simulink model "VDC_TEST_VERNIS"  (R2023b)
settings: Solver=FixedStepAuto  StartTime=0.0  StopTime=10.0  RelTol=1e-3
libraries: simulink x3
settings Model: Creator=no  LastModifiedBy=no
settings OptimizationCC: DefaultParameterBehavior=Inlined
settings RTWCC: Description=INTECRIO Real-Time Target  SystemTargetFile=irt.tlc  TemplateMakefile=irt_default_tmf
settings STFCustomTargetCC: UtilityFuncGeneration=Shared location  MatFileLogging=on  GRTInterface=on  SystemTargetFile=irt.tlc
settings GRTTargetCC: UtilityFuncGeneration=Shared location  ParMdlRefBuildCompliant=off  CompOptLevelCompliant=off  ConcurrentExecutionCompliant=off  CombineOutputUpdateFcns=off  CPPClassGenCompliant=off  GRTInterface=on  UseToolchainInfoCompliant=off  GenerateASAP2=on

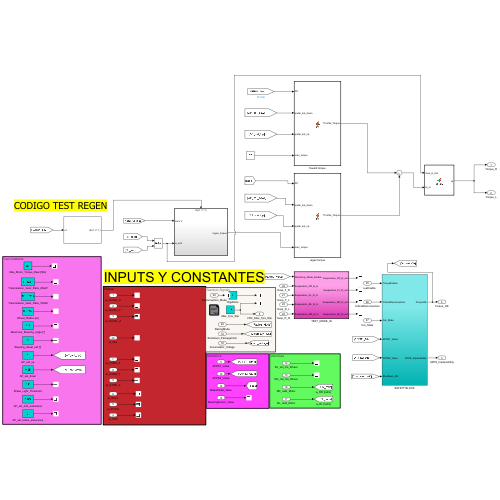
[thumbnail: Simulink's stored preview of the top-level diagram]
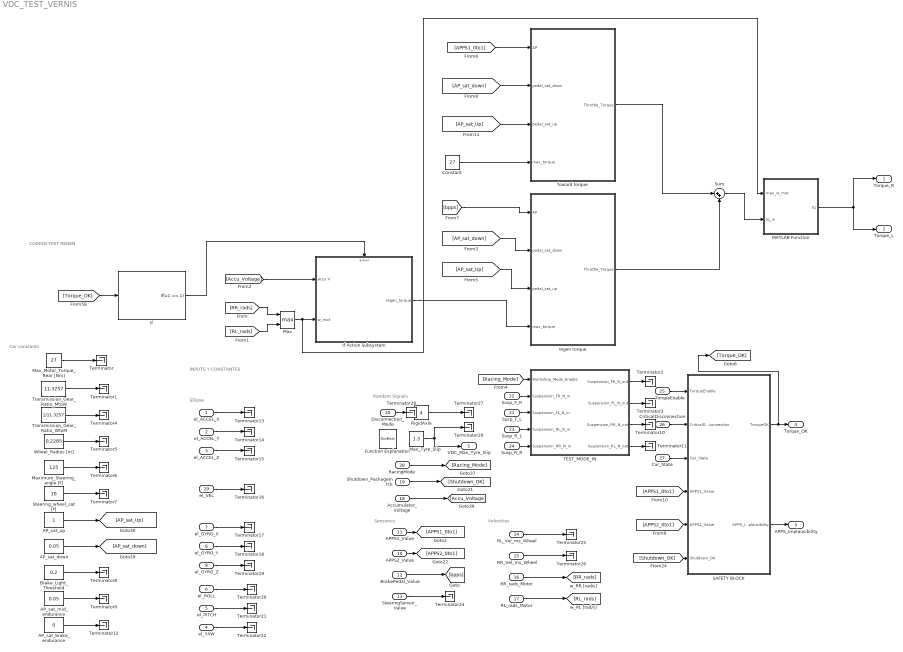
== system VDC_TEST_VERNIS ==
  note: CODIGO TEST REGEN
  note: INPUTS Y CONSTANTES
  note: Ellipse
  note: Sensorics
  note: Velocities
  note: Car constants
  note: Random Signals
  el_ACCEL_X : Inport
  el_ACCEL_Y : Inport  Port=2
  el_ACCEL_Z : Inport  Port=3
  el_YAW : Inport  Port=4
  el_PITCH : Inport  Port=5
  el_ROLL : Inport  Port=6
  el_GYRO_X : Inport  Port=7
  el_GYRO_Y : Inport  Port=8
  el_GYRO_Z : Inport  Port=9
  APPS2_Value : Inport  Port=10
  APPS1_Value : Inport  Port=11
  BrakePedal_Value : Inport  Port=12
  SteeringSensor_Value : Inport  Port=13
  RL_Vel_ms_Wheel : Inport  Port=14
  RR_Vel_ms_Wheel : Inport  Port=15
  RR_rads_Motor : Inport  Port=16
  RL_rads_Motor : Inport  Port=17
  Accumulator_Voltage : Inport  Port=18
  Shutdown_PackageIntck : Inport  Port=19
  Disconnection_Mode : Inport  Port=20
  Susp_F_L : Inport  Port=21
  Susp_F_R : Inport  Port=22
  Susp_R_L : Inport  Port=23
  Susp_R_R : Inport  Port=24
  TorqueEnable : Inport  Port=25
  CriticalDisconnection : Inport  Port=26
  Car_State : Inport  Port=27
  RacingMode : Inport  Port=28
  el_VEL : Inport  Port=29
  AP_sat_brake_endurance : Constant  Value=0
  AP_sat_down : Constant  Value=0.05
  AP_sat_mid_endurance : Constant  Value=0.05
  AP_sat_up : Constant
  Brake_Light_Threshold : Constant  Value=0.2
  Constant : Constant  Value=27
  Function Explanation : simulink/Model-Wide Utilities/DocBlock  DocumentType=Text
      content=|
      | Comparing the speed of the Ellipse and the speed of the Wheels, we can
      | determine the % of deviation between both (which is the slip). With
      | calculations from the Tyres & Performance Department, we know that the
      | maximum optimal slip in a STRAIGHT line is 15%. Therefore (using the Magic
      | Formula), we can determine the maximum X-Force permissible by the Wheels
      | with that % of slip (which is the constant Max_Fx_Tyre, input
      | of Rigid Axle).
      |
      | With that and the radius of the Wheels, we can calculate the maximum
      | Torque for it to stop slipping.
  If : If  IfExpression=u1 == 1  ShowElse=off
  If Action Subsystem : Subsystem  TreatAsAtomicUnit=on
  MATLAB Function : MATLAB Function  TreatAsAtomicUnit=on
  Max : MinMax  Function=max  Inputs=2
  Max_Motor_Torque_Rear [Nm] : Constant  Value=27
  Max_Tyre_Slip : Constant  Value=1.3
  Maximum_Steering_angle [º] : Constant  Value=125
  RigidAxle : Constant  Value=4
  SAFETY BLOCK : Subsystem
  Steering_wheel_sat [º] : Constant  Value=10
  Sum : Sum  Inputs=|++
  TEST_MODE_IN : Subsystem  TreatAsAtomicUnit=on
  Terminator{,1..22,24..29} (29 alike) : Terminator
  Transmission_Gear_Ratio_MtoW : Constant  Value=11.3257
  Transmission_Gear_Ratio_WtoM : Constant  Value=1/11.3257
  Wheel_Radius [m] : Constant  Value=0.2285
  foward torque : MATLAB Function  TreatAsAtomicUnit=on
  regen torque : MATLAB Function  TreatAsAtomicUnit=on
  Torque_R : Outport
  Torque_L : Outport  Port=2
  APPS_Implausibility : Outport  Port=3  VectorParamsAs1DForOutWhenUnconnected=off
  Torque_OK : Outport  Port=4  VectorParamsAs1DForOutWhenUnconnected=off
  VDC_Max_Tyre_Slip : Outport  Port=5
  wires:
  SteeringSensor_Value/1 -> Terminator24/1
  APPS1_Value/1 -> [APPS1_0to1]
  BrakePedal_Value/1 -> [bpps]
  APPS2_Value/1 -> [APPS2_0to1]
  Transmission_Gear_Ratio_MtoW/1 -> Terminator1/1
  Transmission_Gear_Ratio_WtoM/1 -> Terminator4/1
  Wheel_Radius [m]/1 -> Terminator5/1
  Max_Motor_Torque_Rear [Nm]/1 -> Terminator/1
  Shutdown_PackageIntck/1 -> [Shutdown_OK]
  Accumulator_Voltage/1 -> [Accu_Voltage]
  Maximum_Steering_angle [º]/1 -> Terminator6/1
  Steering_wheel_sat [º]/1 -> Terminator7/1
  [Racing_Mode] -> TEST_MODE_IN/1(Workshop_Mode_Enable)
  Susp_F_R/1 -> TEST_MODE_IN/2(Suspension_FR_N_in)
  Susp_R_L/1 -> TEST_MODE_IN/4(Suspension_RL_N_in)
  Susp_R_R/1 -> TEST_MODE_IN/5(Suspension_RR_N_in)
  Susp_F_L/1 -> TEST_MODE_IN/3(Suspension_FL_N_in)
  Max_Tyre_Slip/1 -> Terminator29/1, VDC_Max_Tyre_Slip/1
  CriticalDisconnection/1 -> SAFETY BLOCK/2(CriticalDisconnection)
  TorqueEnable/1 -> SAFETY BLOCK/1(TorqueEnable)
  SAFETY BLOCK/1(TorqueOK) -> Torque_OK/1, [Torque_OK]
  [APPS1_0to1] -> SAFETY BLOCK/4(APPS1_Value)
  SAFETY BLOCK/2(APPS_Implausibility) -> APPS_Implausibility/1
  [APPS2_0to1] -> SAFETY BLOCK/5(APPS2_Value)
  [Shutdown_OK] -> SAFETY BLOCK/6(Shutdown_OK)
  Car_State/1 -> SAFETY BLOCK/3(Car_State)
  AP_sat_up/1 -> [AP_sat_Up]
  AP_sat_down/1 -> [AP_sat_down]
  TEST_MODE_IN/2(Suspension_FL_N_out) -> Terminator3/1
  TEST_MODE_IN/4(Suspension_RL_N_out) -> Terminator11/1
  TEST_MODE_IN/3(Suspension_RR_N_out) -> Terminator10/1
  TEST_MODE_IN/1(Suspension_FR_N_out) -> Terminator2/1
  RacingMode/1 -> [Racing_Mode]
  RL_rads_Motor/1 -> [RL_rads]
  RR_rads_Motor/1 -> [RR_rads]
  RR_Vel_ms_Wheel/1 -> Terminator26/1
  RL_Vel_ms_Wheel/1 -> Terminator25/1
  Brake_Light_Threshold/1 -> Terminator8/1
  AP_sat_mid_endurance/1 -> Terminator9/1
  AP_sat_brake_endurance/1 -> Terminator12/1
  RigidAxle/1 -> Terminator27/1
  [Torque_OK] -> If/1
  If/1 -> If Action Subsystem/Action
  [Accu_Voltage] -> If Action Subsystem/1(accu V)
  [RR_rads] -> Max/1
  [RL_rads] -> Max/2
  Max/1 -> MATLAB Function/1(max_w_mot), If Action Subsystem/2(w_mot)
  If Action Subsystem/1(regen_torque) -> regen torque/4(max_torque)
  el_ACCEL_Z/1 -> Terminator15/1
  el_ACCEL_Y/1 -> Terminator14/1
  el_ACCEL_X/1 -> Terminator13/1
  el_VEL/1 -> Terminator16/1
  el_GYRO_Z/1 -> Terminator19/1
  el_GYRO_Y/1 -> Terminator18/1
  el_GYRO_X/1 -> Terminator17/1
  el_PITCH/1 -> Terminator21/1
  el_ROLL/1 -> Terminator20/1
  el_YAW/1 -> Terminator22/1
  Disconnection_Mode/1 -> Terminator28/1
  [APPS1_0to1] -> foward torque/1(AP)
  [bpps] -> regen torque/1(AP)
  [AP_sat_Up] -> regen torque/3(pedal_sat_up)
  [AP_sat_down] -> regen torque/2(pedal_sat_down)
  [AP_sat_down] -> foward torque/2(pedal_sat_down)
  [AP_sat_Up] -> foward torque/3(pedal_sat_up)
  Constant/1 -> foward torque/4(max_torque)
  foward torque/1(Throttle_Torque) -> Sum/1
  regen torque/1(Throttle_Torque) -> Sum/2
  Sum/1 -> MATLAB Function/2(tq_in)
  MATLAB Function/1(tq) -> Torque_L/1, Torque_R/1

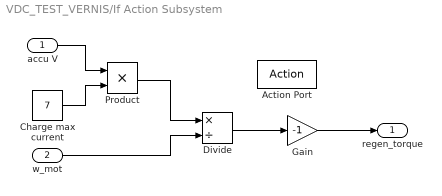
== system VDC_TEST_VERNIS/If Action Subsystem ==
  accu V : Inport
  w_mot : Inport  Port=2
  Action Port : ActionPort  ActionPortLabel=if(u1 == 1)
  Charge max current : Constant  Value=7
  Divide : Product  Inputs=*/
  Gain : Gain  Gain=-1
  Product : Product
  regen_torque : Outport
  wires:
  Gain/1 -> regen_torque/1
  Charge max current/1 -> Product/2
  w_mot/1 -> Divide/2
  Divide/1 -> Gain/1
  accu V/1 -> Product/1
  Product/1 -> Divide/1

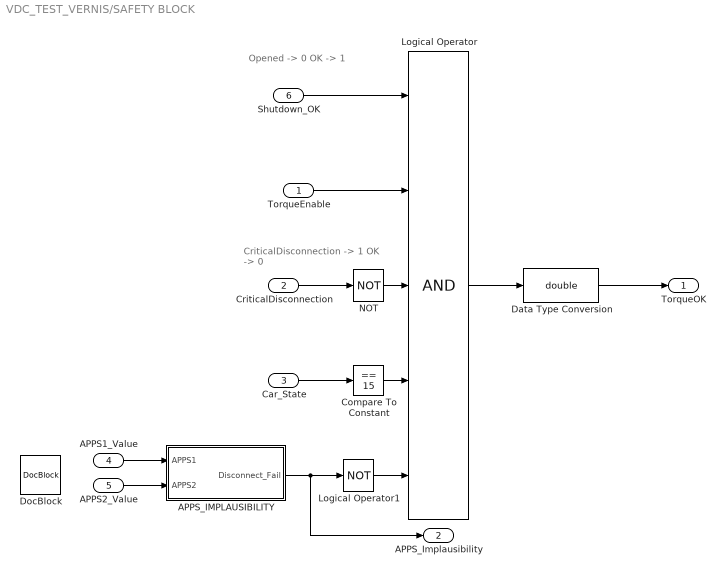
== system VDC_TEST_VERNIS/SAFETY BLOCK ==
  note: CriticalDisconnection -> 1
      | OK -> 0
  note: Opened -> 0
      | OK -> 1
  TorqueEnable : Inport
  CriticalDisconnection : Inport  Port=2
  Car_State : Inport  Port=3
  APPS1_Value : Inport  Port=4
  APPS2_Value : Inport  Port=5
  Shutdown_OK : Inport  Port=6
  APPS_IMPLAUSIBILITY : Subsystem
  Compare To Constant : simulink/Logic and Bit Operations/Compare To Constant  relop===  const=15  OutDataTypeStr=boolean
  Data Type Conversion : DataTypeConversion  OutDataTypeStr=double  SaturateOnIntegerOverflow=off  RndMeth=Floor
  DocBlock : simulink/Model-Wide Utilities/DocBlock  DocumentType=Text
      content=|
      | Formula Student Rules 2024 -> T11.8.8
      |     If an implausibility occurs between the values of the APPSs and
      |     persists for more than 100 ms:
      |     • [EV ONLY] The power to the motor(s) must be immediately shut down
      |     completely. It is not necessary to completely deactivate the TS, the
      |     motor controller(s) shutting down the power to the motor(s) is
      |     sufficient.
      |
      | The 'Number_of_Periods' constant, if there's an Implausability, outputs the error X
      | periods (100ms) after the Implausibility happened (25ms * X = 100ms).
  Logical Operator : Logic  Inputs=5  OutDataTypeStr=boolean
  Logical Operator1 : Logic  Operator=NOT  IconShape=distinctive  AllPortsSameDT=off  OutDataTypeStr=boolean
  NOT : Logic  Operator=NOT  IconShape=distinctive  AllPortsSameDT=off  OutDataTypeStr=boolean
  TorqueOK : Outport  VectorParamsAs1DForOutWhenUnconnected=off
  APPS_Implausibility : Outport  Port=2  VectorParamsAs1DForOutWhenUnconnected=off
  wires:
  Logical Operator/1 -> Data Type Conversion/1
  Car_State/1 -> Compare To Constant/1
  NOT/1 -> Logical Operator/3
  CriticalDisconnection/1 -> NOT/1
  TorqueEnable/1 -> Logical Operator/2
  APPS2_Value/1 -> APPS_IMPLAUSIBILITY/2(APPS2)
  APPS1_Value/1 -> APPS_IMPLAUSIBILITY/1(APPS1)
  APPS_IMPLAUSIBILITY/1(Disconnect_Fail) -> APPS_Implausibility/1, Logical Operator1/1
  Compare To Constant/1 -> Logical Operator/4
  Shutdown_OK/1 -> Logical Operator/1
  Logical Operator1/1 -> Logical Operator/5
  Data Type Conversion/1 -> TorqueOK/1

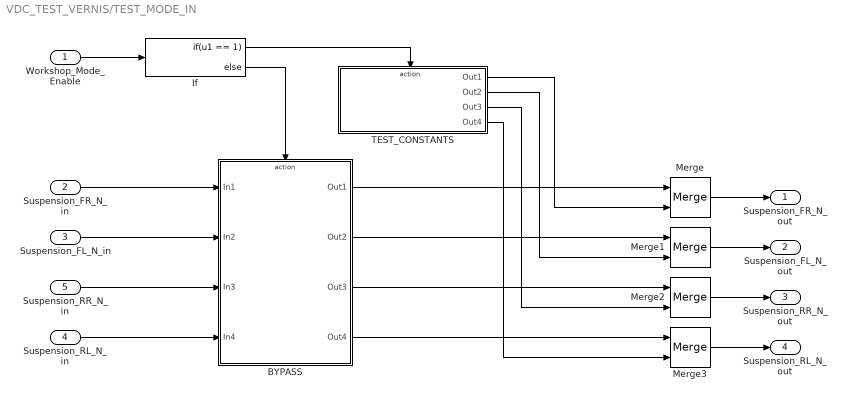
== system VDC_TEST_VERNIS/TEST_MODE_IN ==
  Workshop_Mode_Enable : Inport
  Suspension_FR_N_in : Inport  Port=2
  Suspension_FL_N_in : Inport  Port=3
  Suspension_RL_N_in : Inport  Port=4
  Suspension_RR_N_in : Inport  Port=5
  BYPASS : Subsystem  TreatAsAtomicUnit=on
  If : If  IfExpression=u1 == 1
  Merge{,1..3} (4 alike) : Merge
  TEST_CONSTANTS : Subsystem  TreatAsAtomicUnit=on
  Suspension_FR_N_out : Outport  VectorParamsAs1DForOutWhenUnconnected=off
  Suspension_FL_N_out : Outport  Port=2  VectorParamsAs1DForOutWhenUnconnected=off
  Suspension_RR_N_out : Outport  Port=3  VectorParamsAs1DForOutWhenUnconnected=off
  Suspension_RL_N_out : Outport  Port=4  VectorParamsAs1DForOutWhenUnconnected=off
  wires:
  Suspension_FR_N_in/1 -> BYPASS/1(In1)
  Suspension_FL_N_in/1 -> BYPASS/2(In2)
  Suspension_RR_N_in/1 -> BYPASS/3(In3)
  Suspension_RL_N_in/1 -> BYPASS/4(In4)
  Merge/1 -> Suspension_FR_N_out/1
  Merge1/1 -> Suspension_FL_N_out/1
  Merge2/1 -> Suspension_RR_N_out/1
  Merge3/1 -> Suspension_RL_N_out/1
  BYPASS/1(Out1) -> Merge/1
  BYPASS/2(Out2) -> Merge1/1
  BYPASS/3(Out3) -> Merge2/1
  BYPASS/4(Out4) -> Merge3/1
  Workshop_Mode_Enable/1 -> If/1
  If/2 -> BYPASS/Action
  If/1 -> TEST_CONSTANTS/Action
  TEST_CONSTANTS/4(Out4) -> Merge3/2
  TEST_CONSTANTS/3(Out3) -> Merge2/2
  TEST_CONSTANTS/2(Out2) -> Merge1/2
  TEST_CONSTANTS/1(Out1) -> Merge/2

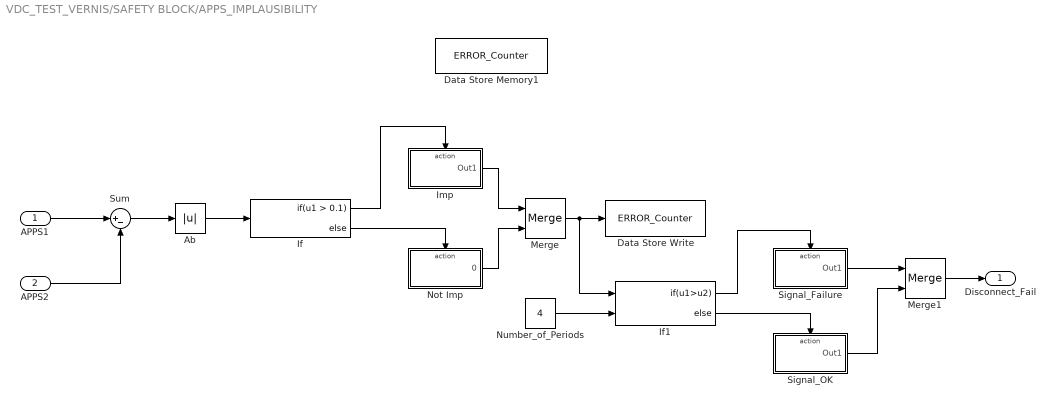
== system VDC_TEST_VERNIS/SAFETY BLOCK/APPS_IMPLAUSIBILITY ==
  APPS1 : Inport
  APPS2 : Inport  Port=2
  Ab : Abs  SaturateOnIntegerOverflow=off
  Data Store Memory1 : DataStoreMemory  DataStoreName=ERROR_Counter  ReadBeforeWriteMsg=warning  WriteAfterWriteMsg=warning  WriteAfterReadMsg=warning  ShowAdditionalParam=off
  Data Store Write : DataStoreWrite  DataStoreName=ERROR_Counter  IndexOptions=Index vector (dialog)  Indices=1  OutputSizes=1
  If : If  IfExpression=u1 > 0.1
  If1 : If  NumInputs=2  IfExpression=u1>u2
  Imp : Subsystem  TreatAsAtomicUnit=on
  Merge : Merge
  Merge1 : Merge
  Not Imp : Subsystem  TreatAsAtomicUnit=on
  Number_of_Periods : Constant  Value=4
  Signal_Failure : Subsystem  TreatAsAtomicUnit=on
  Signal_OK : Subsystem  TreatAsAtomicUnit=on
  Sum : Sum  Inputs=|+-
  Disconnect_Fail : Outport  VectorParamsAs1DForOutWhenUnconnected=off
  wires:
  Number_of_Periods/1 -> If1/2
  Imp/1(Out1) -> Merge/1
  Signal_Failure/1(Out1) -> Merge1/1
  Signal_OK/1(Out1) -> Merge1/2
  Merge1/1 -> Disconnect_Fail/1
  APPS1/1 -> Sum/1
  If/1 -> Imp/Action
  If1/2 -> Signal_OK/Action
  Merge/1 -> Data Store Write/1, If1/1
  If1/1 -> Signal_Failure/Action
  APPS2/1 -> Sum/2
  Ab/1 -> If/1
  If/2 -> Not Imp/Action
  Sum/1 -> Ab/1
  Not Imp/1(0) -> Merge/2

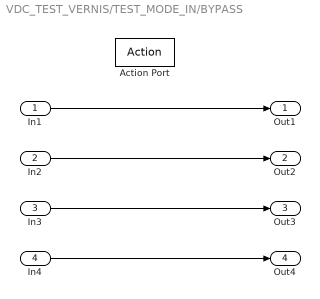
== system VDC_TEST_VERNIS/TEST_MODE_IN/BYPASS ==
  In1 : Inport
  In2 : Inport  Port=2
  In3 : Inport  Port=3
  In4 : Inport  Port=4
  Action Port : ActionPort  ActionPortLabel=else
  Out1 : Outport  VectorParamsAs1DForOutWhenUnconnected=off
  Out2 : Outport  Port=2  VectorParamsAs1DForOutWhenUnconnected=off
  Out3 : Outport  Port=3  VectorParamsAs1DForOutWhenUnconnected=off
  Out4 : Outport  Port=4  VectorParamsAs1DForOutWhenUnconnected=off
  wires:
  In1/1 -> Out1/1
  In2/1 -> Out2/1
  In3/1 -> Out3/1
  In4/1 -> Out4/1

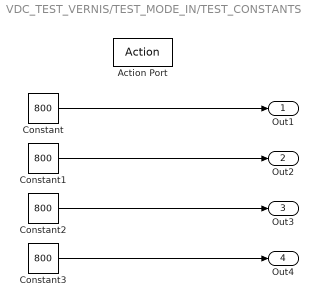
== system VDC_TEST_VERNIS/TEST_MODE_IN/TEST_CONSTANTS ==
  Action Port : ActionPort  ActionPortLabel=if(u1 == 1)
  Constant{,1..3} (4 alike) : Constant  Value=800
  Out1 : Outport  VectorParamsAs1DForOutWhenUnconnected=off
  Out2 : Outport  Port=2  VectorParamsAs1DForOutWhenUnconnected=off
  Out3 : Outport  Port=3  VectorParamsAs1DForOutWhenUnconnected=off
  Out4 : Outport  Port=4  VectorParamsAs1DForOutWhenUnconnected=off
  wires:
  Constant/1 -> Out1/1
  Constant1/1 -> Out2/1
  Constant2/1 -> Out3/1
  Constant3/1 -> Out4/1

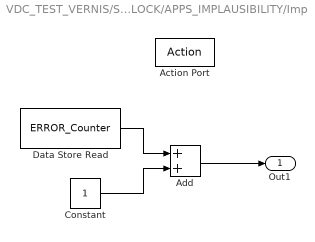
== system VDC_TEST_VERNIS/SAFETY BLOCK/APPS_IMPLAUSIBILITY/Imp ==
  Action Port : ActionPort  ActionPortLabel=if(u1 > 0.1)
  Add : Sum
  Constant : Constant  OutDataTypeStr=boolean
  Data Store Read : DataStoreRead  DataStoreName=ERROR_Counter  IndexOptions=Index vector (dialog)  Indices=1  OutputSizes=1
  Out1 : Outport  VectorParamsAs1DForOutWhenUnconnected=off
  wires:
  Data Store Read/1 -> Add/1
  Constant/1 -> Add/2
  Add/1 -> Out1/1

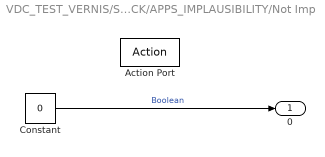
== system VDC_TEST_VERNIS/SAFETY BLOCK/APPS_IMPLAUSIBILITY/Not Imp ==
  Action Port : ActionPort  ActionPortLabel=else
  Constant : Constant  Value=0  OutDataTypeStr=double
  0 : Outport  VectorParamsAs1DForOutWhenUnconnected=off
  wires:
  Constant/1 -> 0/1  "Boolean"

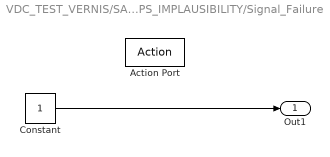
== system VDC_TEST_VERNIS/SAFETY BLOCK/APPS_IMPLAUSIBILITY/Signal_Failure ==
  Action Port : ActionPort  ActionPortLabel=if(u1>u2)
  Constant : Constant
  Out1 : Outport  VectorParamsAs1DForOutWhenUnconnected=off
  wires:
  Constant/1 -> Out1/1

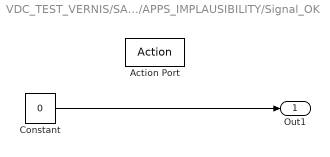
== system VDC_TEST_VERNIS/SAFETY BLOCK/APPS_IMPLAUSIBILITY/Signal_OK ==
  Action Port : ActionPort  ActionPortLabel=else
  Constant : Constant  Value=0
  Out1 : Outport  VectorParamsAs1DForOutWhenUnconnected=off
  wires:
  Constant/1 -> Out1/1

== matlab function VDC_TEST_VERNIS/foward torque ==
  data: Throttle_Torque output; AP input; pedal_sat_down input; pedal_sat_up input; max_torque input
function Throttle_Torque  = TT(AP, pedal_sat_down, pedal_sat_up, max_torque)
    if AP <= pedal_sat_down  
        Throttle_Response = 0;

    elseif AP >= pedal_sat_up % establish the higher deadzone for the throttle pedal
        Throttle_Response = 1;

    else
        Throttle_Response = ((AP - pedal_sat_down) / (pedal_sat_up - pedal_sat_down)); %evaluate for given input
    end
    Throttle_Torque = Throttle_Response * max_torque; % set torque to max output times pedal factor
end

== matlab function VDC_TEST_VERNIS/MATLAB Function ==
  data: max_w_mot input; tq output; tq_in input
function tq = safety(max_w_mot, tq_in)
    if(max_w_mot > 1250 || max_w_mot < 0)
        tq = 0;
        return;
    end
    tq = tq_in;
    return;
end

== matlab function VDC_TEST_VERNIS/regen torque ==
  data: Throttle_Torque output; AP input; pedal_sat_down input; pedal_sat_up input; max_torque input
function Throttle_Torque  = TT(AP, pedal_sat_down, pedal_sat_up, max_torque)
    if AP <= pedal_sat_down
        Throttle_Response = 0;

    elseif AP >= pedal_sat_up % establish the higher deadzone for the throttle pedal
        Throttle_Response = 1;

    else
        Throttle_Response = ((AP - pedal_sat_down) / (pedal_sat_up - pedal_sat_down)); %evaluate for given input
    end
    Throttle_Torque = Throttle_Response * max_torque; % set torque to max output times pedal factor
end
